simulink model "px4_noGPS1"  (R2022a)
settings: Solver=FixedStepDiscrete  StartTime=0.0  StopTime=inf  FixedStep=0.005  MaxStep=0.000005  RelTol=1e-3  EnableMultiTasking=on
InitFcn:
  | I_x = 0.00478;
  | I_y = 0.00502;
  | I_z = 0.00736;
  | m=1;
  | L=0.11667;
undefined symbols (not defined in the file): alt, cog_rad, dev, DiscIntNeverNeededParam, eph, epv, fix_type, lat, lon, m_to_mm, Main, ms_to_cms, pwm_output0, ref_height, ref_lat, ref_lon, SampleTime, satellites_used, time_utc_usec, vel_d_m_s, vel_e_m_s, vel_m_s, vel_n_m_s, vx, vy, vz, x, y, z
libraries: simulink x26, px4uORBlib x5, px4lib x3, etargetslib x1, sensorgpslib x1, slpidlib x1, sharedtransform x1, px4Sensorslib x1
(part 1 of 3)
settings Model: SimulationMode=external  ExtModeTrigDuration=10  Creator=The MathWorks, Inc.  LastModifiedBy=001
settings SolverCC: AlgebraicLoopSolver=TrustRegion  PositivePriorityOrder=on  AutoInsertRateTranBlk=on
settings DataIOCC: LimitDataPoints=on  MaxDataPoints=10000
settings OptimizationCC: BlockReduction=off  EnhancedBackFolding=on  PassReuseOutputArgsAs=Individual arguments  MaxStackSize=64  OptimizeBlockOrder=speed  DifferentSizesBufferReuse=on  OptimizationCustomize=off  EfficientTunableParamExpr=on
settings DebuggingCC: MultiTaskDSMMsg=none  ParameterTunabilityLossMsg=error  UnconnectedInputMsg=warning  UnconnectedOutputMsg=warning  UnconnectedLineMsg=warning  SFMachineParentedDataDiag=warning  ArithmeticOperatorsInVariantConditions=warning
settings HardwareCC: ProdBitPerPointer=32  ProdBitPerSizeT=32  ProdBitPerPtrDiffT=32  ProdLargestAtomicInteger=Long  ProdLargestAtomicFloat=Double  ProdWordSize=32  ProdLongLongMode=on  ProdHWDeviceType=ARM Compatible->ARM Cortex
settings SFSimCC: SimTargetLang=C++
settings RTWCC: SystemTargetFile=ert.tlc  HardwareBoard=PX4 Pixhawk 1  TLCOptions="-aInlineSetEventsForThisBaseRateFcn=TLC_FALSE -aSuppressMultiTaskScheduler=TLC_FALSE  -aRateBasedStepFcn=0"  TemplateMakefile=ert_default_tmf  GenerateReport=on  Toolchain=GNU Tools for PX4 Autopilots  IncludeHyperlinkInReport=on  LaunchReport=on  TargetLang=C++  GenerateTraceInfo=on  GenerateTraceReport=on  GenerateTraceReportSl=on  GenerateTraceReportSf=on  GenerateTraceReportEml=on
settings CodeAppCC: ForceParamTrailComments=on  IgnoreCustomStorageClasses=off  OperatorAnnotations=on  SimulinkDataObjDesc=on  SFDataObjDesc=on  InsertBlockDesc=on
settings ERTTargetCC: SupportContinuousTime=on  SupportNonInlinedSFcns=on  SupportVariableSizeSignals=on  ExtMode=on  ExtModeMexArgs='127.0.0.1' 1 17725

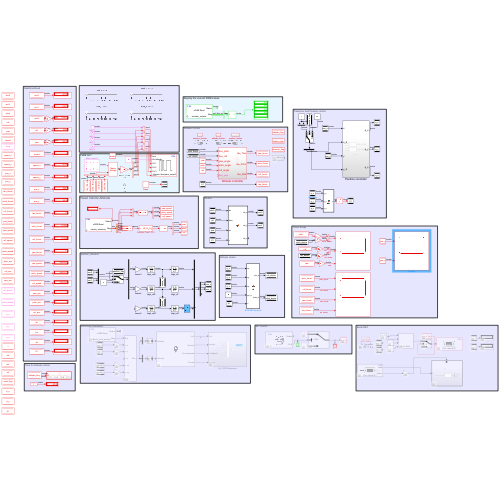
[thumbnail: Simulink's stored preview of the top-level diagram]
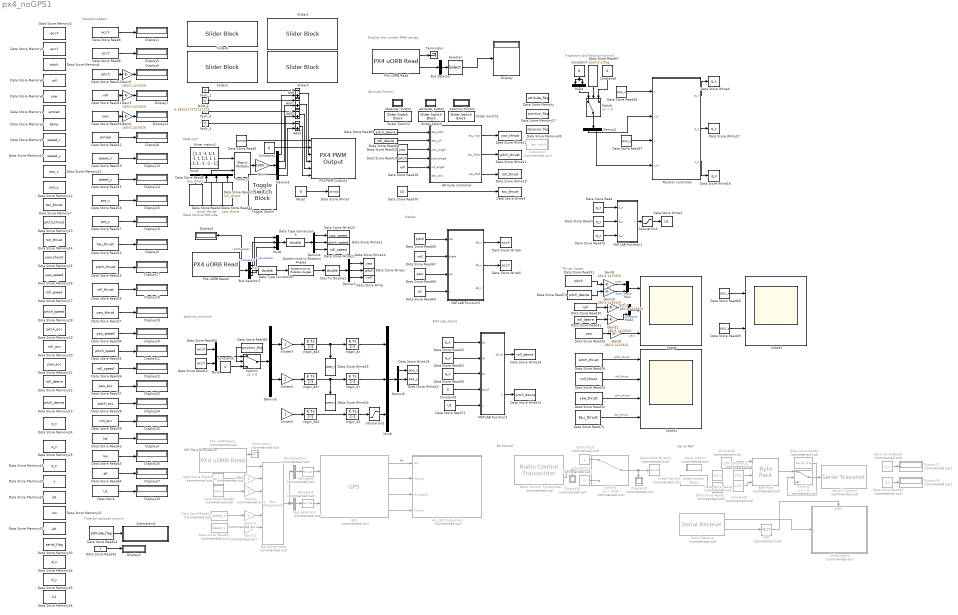
== system px4_noGPS1 ==
  note: Serial R&T
  note: GPS Data Simulation
  note: RC Control
  note: Time for attitude control
  note: position_simulink
  note: Thrust Scope
  note: Attitude Control
  note: DataStoreRead
  note: Display the current PWM values
  note: PWM OUT
  note: Read Vehicle Attitude
  note: Attitude_desire
  note: Trajectory And Position control
  note: GetAcc
  Add{,1..3} (4 alike) : Sum  Inputs=-+  OutDataTypeStr=uint16
  Attitude controller : Subsystem
  Bus Assignment : BusAssignment  Commented=on  AssignedSignals=x,y,z,vx,vy,vz
  Bus Selector : BusSelector  OutputSignals=output  OutputAsBus=on
  Bus Selector1 : BusSelector  Commented=on  OutputSignals=x,y,z  OutputAsBus=on
  Bus Selector2 : BusSelector  OutputSignals=yawspeed,pitchspeed,rollspeed,q
  Bus Selector3 : BusSelector  Commented=on  OutputSignals=vx,vy,vz  OutputAsBus=on
  Byte Pack : etargetslib/Byte Pack  Commented=on  datatypes={'uint8' 'uint8' 'double' 'double'}  byteAlign=1
  Cast To Double1 : DataTypeConversion  OutDataTypeStr=double  SaturateOnIntegerOverflow=off  RndMeth=Floor
  Constant10 : Constant  Commented=on  OutDataTypeStr=boolean
  Constant11 : Constant  Commented=on  Value=0  OutDataTypeStr=boolean
  Constant12 : Constant  Commented=on  Value=10.2  OutDataTypeStr=double
  Constant2 : Constant  Value=0  OutDataTypeStr=boolean
  Constant4 : Constant  Commented=on  Value=10.1  OutDataTypeStr=double
  Constant{5..8} (4 alike) : Constant  Value=0
  Constant9 : Constant  Commented=on  Value=170  OutDataTypeStr=uint8
  "Data Store " : DataStoreRead  DataStoreName=U1  IndexOptions=Index vector (dialog)  Indices=1  OutputSizes=1
  Data Store Memory : DataStoreMemory  DataStoreName=attitude_flag  ReadBeforeWriteMsg=warning  WriteAfterWriteMsg=warning  WriteAfterReadMsg=warning  ShowAdditionalParam=off  OutDataTypeStr=boolean
  Data Store Memory1 : DataStoreMemory  DataStoreName=armed  ReadBeforeWriteMsg=warning  WriteAfterWriteMsg=warning  WriteAfterReadMsg=warning  ShowAdditionalParam=off  OutDataTypeStr=boolean
  Data Store Memory10 : DataStoreMemory  DataStoreName=speed_y  ReadBeforeWriteMsg=warning  WriteAfterWriteMsg=warning  WriteAfterReadMsg=warning  ShowAdditionalParam=off  OutDataTypeStr=double
  Data Store Memory11 : DataStoreMemory  DataStoreName=pos_x  ReadBeforeWriteMsg=warning  WriteAfterWriteMsg=warning  WriteAfterReadMsg=warning  ShowAdditionalParam=off  OutDataTypeStr=double
  Data Store Memory12 : DataStoreMemory  DataStoreName=pos_y  ReadBeforeWriteMsg=warning  WriteAfterWriteMsg=warning  WriteAfterReadMsg=warning  ShowAdditionalParam=off  OutDataTypeStr=double
  Data Store Memory13 : DataStoreMemory  DataStoreName=pitch_thrust  ReadBeforeWriteMsg=warning  WriteAfterWriteMsg=warning  WriteAfterReadMsg=warning  ShowAdditionalParam=off  OutDataTypeStr=double
  Data Store Memory14 : DataStoreMemory  DataStoreName=roll_thrust  ReadBeforeWriteMsg=warning  WriteAfterWriteMsg=warning  WriteAfterReadMsg=warning  ShowAdditionalParam=off  OutDataTypeStr=double
  Data Store Memory15 : DataStoreMemory  DataStoreName=yaw_thrust  ReadBeforeWriteMsg=warning  WriteAfterWriteMsg=warning  WriteAfterReadMsg=warning  ShowAdditionalParam=off  OutDataTypeStr=double
  Data Store Memory16 : DataStoreMemory  DataStoreName=yaw_speed  ReadBeforeWriteMsg=warning  WriteAfterWriteMsg=warning  WriteAfterReadMsg=warning  ShowAdditionalParam=off  OutDataTypeStr=double
  Data Store Memory17 : DataStoreMemory  DataStoreName=roll_speed  ReadBeforeWriteMsg=warning  WriteAfterWriteMsg=warning  WriteAfterReadMsg=warning  ShowAdditionalParam=off  OutDataTypeStr=double
  Data Store Memory18 : DataStoreMemory  DataStoreName=pitch_speed  ReadBeforeWriteMsg=warning  WriteAfterWriteMsg=warning  WriteAfterReadMsg=warning  ShowAdditionalParam=off  OutDataTypeStr=double
  Data Store Memory19 : DataStoreMemory  DataStoreName=pitch_acc  ReadBeforeWriteMsg=warning  WriteAfterWriteMsg=warning  WriteAfterReadMsg=warning  ShowAdditionalParam=off  OutDataTypeStr=double
  Data Store Memory2 : DataStoreMemory  DataStoreName=accX  ReadBeforeWriteMsg=warning  WriteAfterWriteMsg=warning  WriteAfterReadMsg=warning  ShowAdditionalParam=off  OutDataTypeStr=double
  Data Store Memory20 : DataStoreMemory  DataStoreName=roll_acc  ReadBeforeWriteMsg=warning  WriteAfterWriteMsg=warning  WriteAfterReadMsg=warning  ShowAdditionalParam=off  OutDataTypeStr=double
  Data Store Memory21 : DataStoreMemory  DataStoreName=yaw_acc  ReadBeforeWriteMsg=warning  WriteAfterWriteMsg=warning  WriteAfterReadMsg=warning  ShowAdditionalParam=off  OutDataTypeStr=double
  Data Store Memory22 : DataStoreMemory  DataStoreName=roll_desire  ReadBeforeWriteMsg=warning  WriteAfterWriteMsg=warning  WriteAfterReadMsg=warning  ShowAdditionalParam=off  OutDataTypeStr=double
  Data Store Memory23 : DataStoreMemory  DataStoreName=pitch_desire  ReadBeforeWriteMsg=warning  WriteAfterWriteMsg=warning  WriteAfterReadMsg=warning  ShowAdditionalParam=off  OutDataTypeStr=double
  Data Store Memory24 : DataStoreMemory  DataStoreName=q_x  ReadBeforeWriteMsg=warning  WriteAfterWriteMsg=warning  WriteAfterReadMsg=warning  ShowAdditionalParam=off  OutDataTypeStr=double
  Data Store Memory25 : DataStoreMemory  DataStoreName=q_y  ReadBeforeWriteMsg=warning  WriteAfterWriteMsg=warning  WriteAfterReadMsg=warning  ShowAdditionalParam=off  OutDataTypeStr=double
  Data Store Memory26 : DataStoreMemory  DataStoreName=q_z  ReadBeforeWriteMsg=warning  WriteAfterWriteMsg=warning  WriteAfterReadMsg=warning  ShowAdditionalParam=off  OutDataTypeStr=double
  Data Store Memory27 : DataStoreMemory  DataStoreName=position_flag  ReadBeforeWriteMsg=warning  WriteAfterWriteMsg=warning  WriteAfterReadMsg=warning  ShowAdditionalParam=off  OutDataTypeStr=boolean
  Data Store Memory28 : DataStoreMemory  DataStoreName=lat  ReadBeforeWriteMsg=warning  WriteAfterWriteMsg=warning  WriteAfterReadMsg=warning  ShowAdditionalParam=off
  Data Store Memory29 : DataStoreMemory  DataStoreName=t  ReadBeforeWriteMsg=warning  WriteAfterWriteMsg=warning  WriteAfterReadMsg=warning  ShowAdditionalParam=off
  Data Store Memory3 : DataStoreMemory  DataStoreName=accY  ReadBeforeWriteMsg=warning  WriteAfterWriteMsg=warning  WriteAfterReadMsg=warning  ShowAdditionalParam=off  OutDataTypeStr=double
  Data Store Memory30 : DataStoreMemory  DataStoreName=observer_flag  ReadBeforeWriteMsg=warning  WriteAfterWriteMsg=warning  WriteAfterReadMsg=warning  ShowAdditionalParam=off  OutDataTypeStr=boolean
  Data Store Memory31 : DataStoreMemory  DataStoreName=lon  ReadBeforeWriteMsg=warning  WriteAfterWriteMsg=warning  WriteAfterReadMsg=warning  ShowAdditionalParam=off
  Data Store Memory32 : DataStoreMemory  DataStoreName=alt  ReadBeforeWriteMsg=warning  WriteAfterWriteMsg=warning  WriteAfterReadMsg=warning  ShowAdditionalParam=off
  Data Store Memory33 : DataStoreMemory  DataStoreName=serial_flag  ReadBeforeWriteMsg=warning  WriteAfterWriteMsg=warning  WriteAfterReadMsg=warning  ShowAdditionalParam=off
  Data Store Memory34 : DataStoreMemory  DataStoreName=d_x  ReadBeforeWriteMsg=warning  WriteAfterWriteMsg=warning  WriteAfterReadMsg=warning  ShowAdditionalParam=off
  Data Store Memory35 : DataStoreMemory  DataStoreName=d_y  ReadBeforeWriteMsg=warning  WriteAfterWriteMsg=warning  WriteAfterReadMsg=warning  ShowAdditionalParam=off
  Data Store Memory36 : DataStoreMemory  DataStoreName=U1  ReadBeforeWriteMsg=warning  WriteAfterWriteMsg=warning  WriteAfterReadMsg=warning  ShowAdditionalParam=off
  Data Store Memory4 : DataStoreMemory  DataStoreName=pitch  ReadBeforeWriteMsg=warning  WriteAfterWriteMsg=warning  WriteAfterReadMsg=warning  ShowAdditionalParam=off  OutDataTypeStr=double
  Data Store Memory5 : DataStoreMemory  DataStoreName=temp  ReadBeforeWriteMsg=warning  WriteAfterWriteMsg=warning  WriteAfterReadMsg=warning  ShowAdditionalParam=off  OutDataTypeStr=double  Dimensions=5
  Data Store Memory6 : DataStoreMemory  DataStoreName=roll  ReadBeforeWriteMsg=warning  WriteAfterWriteMsg=warning  WriteAfterReadMsg=warning  ShowAdditionalParam=off  OutDataTypeStr=double
  Data Store Memory7 : DataStoreMemory  DataStoreName=tau_thrust  ReadBeforeWriteMsg=warning  WriteAfterWriteMsg=warning  WriteAfterReadMsg=warning  ShowAdditionalParam=off  OutDataTypeStr=double
  Data Store Memory8 : DataStoreMemory  DataStoreName=yaw  ReadBeforeWriteMsg=warning  WriteAfterWriteMsg=warning  WriteAfterReadMsg=warning  ShowAdditionalParam=off  OutDataTypeStr=double
  Data Store Memory9 : DataStoreMemory  DataStoreName=speed_x  ReadBeforeWriteMsg=warning  WriteAfterWriteMsg=warning  WriteAfterReadMsg=warning  ShowAdditionalParam=off  OutDataTypeStr=double
  Data Store Read : DataStoreRead  DataStoreName=q_x  IndexOptions=Index vector (dialog)  Indices=1  OutputSizes=1
  Data Store Read1 : DataStoreRead  Commented=on  DataStoreName=pos_x  IndexOptions=Index vector (dialog)  Indices=1  OutputSizes=1
  Data Store Read{10,14,31,58} (4 alike) : DataStoreRead  DataStoreName=pitch  IndexOptions=Index vector (dialog)  Indices=1  OutputSizes=1
  Data Store Read{11,18,30,67} (4 alike) : DataStoreRead  DataStoreName=roll  IndexOptions=Index vector (dialog)  Indices=1  OutputSizes=1
  Data Store Read12 : DataStoreRead  DataStoreName=armed  IndexOptions=Index vector (dialog)  Indices=1  OutputSizes=1
  Data Store Read13 : DataStoreRead  DataStoreName=tau_thrust  IndexOptions=Index vector (dialog)  Indices=1  OutputSizes=1
  Data Store Read15 : DataStoreRead  DataStoreName=speed_y  IndexOptions=Index vector (dialog)  Indices=1  OutputSizes=1
  Data Store Read16 : DataStoreRead  DataStoreName=pos_x  IndexOptions=Index vector (dialog)  Indices=1  OutputSizes=1
  Data Store Read17 : DataStoreRead  DataStoreName=pos_y  IndexOptions=Index vector (dialog)  Indices=1  OutputSizes=1
  Data Store Read19 : DataStoreRead  DataStoreName=speed_x  IndexOptions=Index vector (dialog)  Indices=1  OutputSizes=1
  Data Store Read2 : DataStoreRead  Commented=on  DataStoreName=pos_y  IndexOptions=Index vector (dialog)  Indices=1  OutputSizes=1
  Data Store Read{20,24,33,66} (4 alike) : DataStoreRead  DataStoreName=yaw  IndexOptions=Index vector (dialog)  Indices=1  OutputSizes=1
  Data Store Read21 : DataStoreRead  DataStoreName=roll_thrust  IndexOptions=Index vector (dialog)  Indices=1  OutputSizes=1
  Data Store Read22 : DataStoreRead  DataStoreName=yaw_thrust  IndexOptions=Index vector (dialog)  Indices=1  OutputSizes=1
  Data Store Read23 : DataStoreRead  DataStoreName=pitch_thrust  IndexOptions=Index vector (dialog)  Indices=1  OutputSizes=1
  Data Store Read25 : DataStoreRead  DataStoreName=pitch_thrust  IndexOptions=Index vector (dialog)  Indices=1  OutputSizes=1
  Data Store Read26 : DataStoreRead  DataStoreName=roll_thrust  IndexOptions=Index vector (dialog)  Indices=1  OutputSizes=1
  Data Store Read27 : DataStoreRead  DataStoreName=yaw_thrust  IndexOptions=Index vector (dialog)  Indices=1  OutputSizes=1
  Data Store Read28 : DataStoreRead  DataStoreName=pitch_thrust  IndexOptions=Index vector (dialog)  Indices=1  OutputSizes=1
  Data Store Read29 : DataStoreRead  DataStoreName=roll_thrust  IndexOptions=Index vector (dialog)  Indices=1  OutputSizes=1
  Data Store Read3 : DataStoreRead  DataStoreName=tau_thrust  IndexOptions=Index vector (dialog)  Indices=1  OutputSizes=1
  Data Store Read32 : DataStoreRead  DataStoreName=yaw_thrust  IndexOptions=Index vector (dialog)  Indices=1  OutputSizes=1
  Data Store Read34 : DataStoreRead  DataStoreName=yaw_speed  IndexOptions=Index vector (dialog)  Indices=1  OutputSizes=1
  Data Store Read35 : DataStoreRead  DataStoreName=pitch_speed  IndexOptions=Index vector (dialog)  Indices=1  OutputSizes=1
  Data Store Read36 : DataStoreRead  DataStoreName=roll_speed  IndexOptions=Index vector (dialog)  Indices=1  OutputSizes=1
  Data Store Read37 : DataStoreRead  DataStoreName=yaw_acc  IndexOptions=Index vector (dialog)  Indices=1  OutputSizes=1
  Data Store Read38 : DataStoreRead  DataStoreName=pitch_acc  IndexOptions=Index vector (dialog)  Indices=1  OutputSizes=1
  Data Store Read39 : DataStoreRead  DataStoreName=roll_acc  IndexOptions=Index vector (dialog)  Indices=1  OutputSizes=1
  Data Store Read4 : DataStoreRead  Commented=on  DataStoreName=serial_flag  IndexOptions=Index vector (dialog)  Indices=1  OutputSizes=1
  Data Store Read40 : DataStoreRead  Commented=on  DataStoreName=d_y  IndexOptions=Index vector (dialog)  Indices=1  OutputSizes=1
  Data Store Read41 : DataStoreRead  DataStoreName=roll_desire  IndexOptions=Index vector (dialog)  Indices=1  OutputSizes=1
  Data Store Read42 : DataStoreRead  DataStoreName=lat  IndexOptions=Index vector (dialog)  Indices=1  OutputSizes=1
  Data Store Read43 : DataStoreRead  DataStoreName=lon  IndexOptions=Index vector (dialog)  Indices=1  OutputSizes=1
  Data Store Read44 : DataStoreRead  DataStoreName=alt  IndexOptions=Index vector (dialog)  Indices=1  OutputSizes=1
  Data Store Read45 : DataStoreRead  DataStoreName=q_x  IndexOptions=Index vector (dialog)  Indices=1  OutputSizes=1
  Data Store Read46 : DataStoreRead  DataStoreName=pos_x  IndexOptions=Index vector (dialog)  Indices=1  OutputSizes=1
  Data Store Read47 : DataStoreRead  DataStoreName=pos_y  IndexOptions=Index vector (dialog)  Indices=1  OutputSizes=1
  Data Store Read48 : DataStoreRead  DataStoreName=pos_x  IndexOptions=Index vector (dialog)  Indices=1  OutputSizes=1
  Data Store Read49 : DataStoreRead  DataStoreName=pos_y  IndexOptions=Index vector (dialog)  Indices=1  OutputSizes=1
  Data Store Read5 : DataStoreRead  Commented=on  DataStoreName=d_x  IndexOptions=Index vector (dialog)  Indices=1  OutputSizes=1
  Data Store Read50 : DataStoreRead  DataStoreName=accX  IndexOptions=Index vector (dialog)  Indices=1  OutputSizes=1
  Data Store Read51 : DataStoreRead  DataStoreName=accY  IndexOptions=Index vector (dialog)  Indices=1  OutputSizes=1
  Data Store Read52 : DataStoreRead  DataStoreName=q_y  IndexOptions=Index vector (dialog)  Indices=1  OutputSizes=1
  Data Store Read53 : DataStoreRead  DataStoreName=position_flag  IndexOptions=Index vector (dialog)  Indices=1  OutputSizes=1
  Data Store Read54 : DataStoreRead  DataStoreName=attitude_flag  IndexOptions=Index vector (dialog)  Indices=1  OutputSizes=1
  Data Store Read55 : DataStoreRead  DataStoreName=t  IndexOptions=Index vector (dialog)  Indices=1  OutputSizes=1
  Data Store Read56 : DataStoreRead  DataStoreName=q_z  IndexOptions=Index vector (dialog)  Indices=1  OutputSizes=1
  Data Store Read57 : DataStoreRead  DataStoreName=position_flag  IndexOptions=Index vector (dialog)  Indices=1  OutputSizes=1
  Data Store Read59 : DataStoreRead  Commented=on  DataStoreName=pos_x  IndexOptions=Index vector (dialog)  Indices=1  OutputSizes=1
  Data Store Read6 : DataStoreRead  DataStoreName=armed  IndexOptions=Index vector (dialog)  Indices=1  OutputSizes=1
  Data Store Read60 : DataStoreRead  Commented=on  DataStoreName=pos_y  IndexOptions=Index vector (dialog)  Indices=1  OutputSizes=1
  Data Store Read61 : DataStoreRead  Commented=on  DataStoreName=speed_x  IndexOptions=Index vector (dialog)  Indices=1  OutputSizes=1
  Data Store Read62 : DataStoreRead  Commented=on  DataStoreName=speed_y  IndexOptions=Index vector (dialog)  Indices=1  OutputSizes=1
  Data Store Read63 : DataStoreRead  DataStoreName=U1  IndexOptions=Index vector (dialog)  Indices=1  OutputSizes=1
  Data Store Read68 : DataStoreRead  DataStoreName=roll_desire  IndexOptions=Index vector (dialog)  Indices=1  OutputSizes=1
  Data Store Read69 : DataStoreRead  DataStoreName=pitch_desire  IndexOptions=Index vector (dialog)  Indices=1  OutputSizes=1
  Data Store Read7 : DataStoreRead  DataStoreName=q_y  IndexOptions=Index vector (dialog)  Indices=1  OutputSizes=1
  Data Store Read70 : DataStoreRead  DataStoreName=U1  IndexOptions=Index vector (dialog)  Indices=1  OutputSizes=1
  Data Store Read71 : DataStoreRead  DataStoreName=U1  IndexOptions=Index vector (dialog)  Indices=1  OutputSizes=1
  Data Store Read73 : DataStoreRead  DataStoreName=tau_thrust  IndexOptions=Index vector (dialog)  Indices=1  OutputSizes=1
  Data Store Read74 : DataStoreRead  DataStoreName=pitch_desire  IndexOptions=Index vector (dialog)  Indices=1  OutputSizes=1
  Data Store Read75 : DataStoreRead  DataStoreName=q_z  IndexOptions=Index vector (dialog)  Indices=1  OutputSizes=1
  Data Store Read8 : DataStoreRead  DataStoreName=accX  IndexOptions=Index vector (dialog)  Indices=1  OutputSizes=1
  Data Store Read9 : DataStoreRead  DataStoreName=accY  IndexOptions=Index vector (dialog)  Indices=1  OutputSizes=1
  Data Store Write : DataStoreWrite  DataStoreName=roll  IndexOptions=Index vector (dialog)  Indices=1  OutputSizes=1
  Data Store Write1 : DataStoreWrite  DataStoreName=pitch  IndexOptions=Index vector (dialog)  Indices=1  OutputSizes=1
  Data Store Write10 : DataStoreWrite  DataStoreName=yaw  IndexOptions=Index vector (dialog)  Indices=1  OutputSizes=1
  Data Store Write11 : DataStoreWrite  DataStoreName=yaw_thrust  IndexOptions=Index vector (dialog)  Indices=1  OutputSizes=1
  Data Store Write12 : DataStoreWrite  DataStoreName=pitch_thrust  IndexOptions=Index vector (dialog)  Indices=1  OutputSizes=1
  Data Store Write13 : DataStoreWrite  DataStoreName=roll_thrust  IndexOptions=Index vector (dialog)  Indices=1  OutputSizes=1
  Data Store Write14 : DataStoreWrite  DataStoreName=roll_desire  IndexOptions=Index vector (dialog)  Indices=1  OutputSizes=1
  Data Store Write15 : DataStoreWrite  DataStoreName=pitch_desire  IndexOptions=Index vector (dialog)  Indices=1  OutputSizes=1
  Data Store Write16 : DataStoreWrite  Commented=on  DataStoreName=armed  IndexOptions=Index vector (dialog)  Indices=1  OutputSizes=1
  Data Store Write17 : DataStoreWrite  DataStoreName=q_y  IndexOptions=Index vector (dialog)  Indices=1  OutputSizes=1
  Data Store Write18 : DataStoreWrite  DataStoreName=q_z  IndexOptions=Index vector (dialog)  Indices=1  OutputSizes=1
  Data Store Write19 : DataStoreWrite  DataStoreName=pos_x  IndexOptions=Index vector (dialog)  Indices=1  OutputSizes=1
  Data Store Write2 : DataStoreWrite  DataStoreName=U1  IndexOptions=Index vector (dialog)  Indices=1  OutputSizes=1
  Data Store Write20 : DataStoreWrite  DataStoreName=yaw_speed  IndexOptions=Index vector (dialog)  Indices=1  OutputSizes=1
  Data Store Write21 : DataStoreWrite  DataStoreName=pitch_speed  IndexOptions=Index vector (dialog)  Indices=1  OutputSizes=1
  Data Store Write22 : DataStoreWrite  DataStoreName=roll_speed  IndexOptions=Index vector (dialog)  Indices=1  OutputSizes=1
  Data Store Write23 : DataStoreWrite  DataStoreName=pos_y  IndexOptions=Index vector (dialog)  Indices=1  OutputSizes=1
  Data Store Write24 : DataStoreWrite  DataStoreName=speed_y  IndexOptions=Index vector (dialog)  Indices=1  OutputSizes=1
  Data Store Write25 : DataStoreWrite  DataStoreName=speed_x  IndexOptions=Index vector (dialog)  Indices=1  OutputSizes=1
  Data Store Write4 : DataStoreWrite  DataStoreName=q_x  IndexOptions=Index vector (dialog)  Indices=1  OutputSizes=1
  Data Store Write5 : DataStoreWrite  DataStoreName=accY  IndexOptions=Index vector (dialog)  Indices=1  OutputSizes=1
  Data Store Write6 : DataStoreWrite  DataStoreName=accX  IndexOptions=Index vector (dialog)  Indices=1  OutputSizes=1
  Data Store Write7 : DataStoreWrite  DataStoreName=armed  IndexOptions=Index vector (dialog)  Indices=1  OutputSizes=1
  Data Store Write9 : DataStoreWrite  DataStoreName=tau_thrust  IndexOptions=Index vector (dialog)  Indices=1  OutputSizes=1
  Data Type Conversion1 : DataTypeConversion  OutDataTypeStr=double  SaturateOnIntegerOverflow=off  RndMeth=Floor
  Data Type Conversion3 : DataTypeConversion  OutDataTypeStr=double  SaturateOnIntegerOverflow=off  RndMeth=Floor
  Demux1 : Demux  Outputs=3
  Demux2 : Demux  Outputs=2
  Demux3 : Demux
  Demux4 : Demux  Outputs=3
  Demux5 : Demux  Outputs=2
  Demux6 : Demux  Outputs=3
  Display{,1..9,12..27,30} (27 alike) : Display
  Display{10..11,28..29} (4 alike) : Display  Commented=on
  GPS : sensorgpslib/GPS  Commented=on  DispRefFrame=NED  PositionInputFormat=Local  ReferenceLocation=[ref_lat ref_lon ref_height]  HorizontalPositionAccuracy=0.01  VerticalPositionAccuracy=0.01  VelocityAccuracy=0.01  DecayFactor=0.999  SeedDouble=67  SimulateUsing=Interpreted execution
      settings: SourceProductBaseCode=TF,NV,UV
  Gain{,12..14} (4 alike) : Gain  Commented=on  OutDataTypeStr=single
  Gain{3,5..11} (8 alike) : Gain  Gain=180/3.1415926
  Gain4 : Gain  Gain=1000  OutDataTypeStr=uint16
  HIL_GPS Subsystem : Subsystem  Commented=on
  Intgrt_dX : DiscreteIntegrator  gainval=1  SampleTime=-1  ICPrevOutput=DiscIntNeverNeededParam  ICPrevScaledInput=DiscIntNeverNeededParam
  Intgrt_dY : DiscreteIntegrator  gainval=1  SampleTime=-1  ICPrevOutput=DiscIntNeverNeededParam  ICPrevScaledInput=DiscIntNeverNeededParam
  Intgrt_dZ : DiscreteIntegrator  gainval=1  SampleTime=-1  LowerSaturationLimit=0  ICPrevOutput=DiscIntNeverNeededParam  ICPrevScaledInput=DiscIntNeverNeededParam
  Intgrt_ddX : DiscreteIntegrator  gainval=1  SampleTime=-1  ICPrevOutput=DiscIntNeverNeededParam  ICPrevScaledInput=DiscIntNeverNeededParam
  Intgrt_ddY : DiscreteIntegrator  gainval=1  SampleTime=-1  ICPrevOutput=DiscIntNeverNeededParam  ICPrevScaledInput=DiscIntNeverNeededParam
  Intgrt_ddZ : DiscreteIntegrator  gainval=1  SampleTime=-1  ICPrevOutput=DiscIntNeverNeededParam  ICPrevScaledInput=DiscIntNeverNeededParam
  MATLAB Function1 : MATLAB Function  TreatAsAtomicUnit=on
  MATLAB Function3 : MATLAB Function  TreatAsAtomicUnit=on
  MATLAB Function5 : MATLAB Function  TreatAsAtomicUnit=on
  Mixer matrix1 : Constant  Value=[1 1 -1 1;1 -1 1 1;1 1 1 -1;1 -1 -1 -1]  OutDataTypeStr=Inherit: Inherit via back propagation
  Mux{,2,4..5} (4 alike) : Mux  Inputs=2
  Mux3 : Mux
  Mux6 : Mux  Inputs=3
  Mux8 : Mux  Inputs=3
  NOT : Logic  Commented=on  Operator=NOT  IconShape=distinctive  AllPortsSameDT=off  OutDataTypeStr=boolean
  PX4 PWM Output1 : px4lib/PX4 PWM Output  pwmDevice=Main (/dev/pwm_output0)  pwmChannel1_=on  pwmChannel2_=on  pwmChannel3_=on  pwmChannel4_=on  pwmChannel5_=off  pwmChannel6_=off  pwmChannel7_=off  pwmChannel8_=off  forceTerminateFailsafe=off  outputErrorStatus=off
      settings: SourceProductBaseCode=PX4AUTOPILOTS
  PX4 uORB Read : px4uORBlib/PX4 uORB Read  uORBTopic=actuator_outputs  selectInstance=actuator_outputs  SampleTime=0.01  BlockingMode=off  BlockTimeout=1e-3
      settings: SourceProductBaseCode=PX4AUTOPILOTS
  PX4 uORB Read1 : px4uORBlib/PX4 uORB Read  Commented=on  uORBTopic=vehicle_local_position  selectInstance=vehicle_local_position  SampleTime=-1  BlockingMode=off  BlockTimeout=1e-3
      settings: SourceProductBaseCode=PX4AUTOPILOTS
  PX4 uORB Read2 : px4uORBlib/PX4 uORB Read  uORBTopic=vehicle_odometry  selectInstance=vehicle_odometry  SampleTime=0.005  BlockingMode=off  BlockTimeout=1e-3
      settings: SourceProductBaseCode=PX4AUTOPILOTS
  Position controller : Subsystem
  Product2 : Product  Multiplication=Matrix(*)  RndMeth=Zero
  Quaternions to Rotation Angles : sharedtransform/Quaternions to Rotation Angles  rotationOrder=ZYX  aMode=aMode
      settings: SourceProductBaseCode=AE,PW,DR,MT,VE
  Radio Control Transmitter : px4Sensorslib/Radio Control Transmitter  Commented=on  channel1=off  channel2=off  channel3=off  channel4=off  channel5=off  channel6=off  channel7=off  channel8=on  channel_count=off  rssi=off  rc_input_source=off  timestamp_last_signal=off  time_stamp=off  sampleTime=0.005  BlockingMode=off  BlockTimeout=5
      settings: SourceProductBaseCode=PX4AUTOPILOTS
  Reset : Constant  Value=0  OutDataTypeStr=boolean  SampleTime=-1
      settings: OpenFcn=|
      | if strcmp('0',get_param(gcb, 'Value'))                        set_param(gcb, 'Value', '1');
      | else
      |             set_param(gcb, 'Value', '0');
      | end
  Reshape1 : Reshape  Commented=on  OutputDimensionality=Row vector (2-D)
  Reshape3 : Reshape  Commented=on  OutputDimensionality=Row vector (2-D)
  Saturation1 : Saturate  UpperLimit=inf  LowerLimit=0
  Saturation2 : Saturate  UpperLimit=1.5  LowerLimit=1
  Scope : Scope  NumInputPorts=3
  Scope1 : Scope  NumInputPorts=4
  Scope2 : Scope  NumInputPorts=2
  Selector : Selector  InputPortWidth=16  IndexOptions=Select all  Indices=[1 4]  OutputSizes=1
  Serial Receive : px4lib/Serial Receive  Commented=on  SCIModule=/dev/ttyS1  DataType=uint8  DataLength=36  OutputStatus=on  SampleTime=-1  BlockingMode=off  PartialData=off  Timeout=5
      settings: SourceProductBaseCode=PX4AUTOPILOTS
  Serial Transmit : px4lib/Serial Transmit  Commented=on  SCIModule=/dev/ttyS1
      settings: SourceProductBaseCode=PX4AUTOPILOTS
  Slider Switch : SliderSwitchBlock
      settings: Values={{'Off', 'On'}, [0 1]}
  Slider Switch1 : SliderSwitchBlock
      settings: Values={{'Off', 'On'}, [0 1]}
  Slider Switch2 : SliderSwitchBlock
      settings: Values={{'Off', 'On'}, [0 1]}
  Slider Switch3 : SliderSwitchBlock  Commented=on
      settings: Values={{'Off', 'On'}, [0 1]}
  Slider{1..3,6} (4 alike) : SliderBlock  ScaleMax=200
  Subsystem : Subsystem  Commented=on
  Subsystem1 : Subsystem
  Subsystem2 : Subsystem  Commented=on
  Switch : Switch  Criteria=u2 > Threshold  SaturateOnIntegerOverflow=off  InputSameDT=off
  Switch1 : Switch  Criteria=u2 > Threshold  SaturateOnIntegerOverflow=off  InputSameDT=off
  Switch2 : Switch  Commented=on  Criteria=u2 > Threshold  SaturateOnIntegerOverflow=off  InputSameDT=off
  Switch3 : Switch  Commented=on  Criteria=u2 > Threshold  Threshold=1500  SaturateOnIntegerOverflow=off  InputSameDT=off
  Terminator : Terminator
  Terminator1 : Terminator  Commented=on
  Toggle Switch : ToggleSwitchBlock
      settings: Values={{'Off', 'On'}, [0 1]}
  attitude_button : Subsystem
  fault_1 : Constant  Value=0
  fault_2 : Constant  Value=0.3835227272727273
  fault_3 : Constant  Value=0
  fault_4 : Constant  Value=0
  observer_button : Subsystem
  position_button : Subsystem
  serial_button : Subsystem  Commented=on
  slower3 : Gain
  slower4 : Gain
  slower5 : Gain
  wires:
  PX4 uORB Read/1 -> Terminator/1
  PX4 uORB Read/2 -> Bus Selector/1
  Bus Selector/1 -> Selector/1
  Selector/1 -> Display/1
  PX4 uORB Read2/1 -> Display2/1
  Quaternions to Rotation Angles/1 -> Cast To Double1/1
  Data Type Conversion1/1 -> Quaternions to Rotation Angles/1
  Bus Selector2/4 -> Data Type Conversion1/1  "<q>"
  PX4 uORB Read2/2 -> Bus Selector2/1
  Demux1/3 -> Data Store Write/1
  Demux1/2 -> Data Store Write1/1
  Cast To Double1/1 -> Demux1/1
  Data Store Read8/1 -> Display1/1
  Data Store Read9/1 -> Display5/1
  Data Store Read12/1 -> Display8/1
  Data Store Read19/1 -> Display13/1
  Data Store Read16/1 -> Display15/1
  Data Store Read17/1 -> Display16/1
  Data Store Read15/1 -> Display14/1
  Data Store Read13/1 -> Display9/1
  Mux3/1 -> Product2/2
  Product2/1 -> Gain4/1
  Gain4/1 -> Demux3/1
  Data Store Read3/1 -> Mux3/1
  Data Store Read6/1 -> PX4 PWM Output1/1
  Data Store Read11/1 -> Gain3/1
  Gain3/1 -> Display7/1
  Data Store Read10/1 -> Gain5/1
  Gain5/1 -> Display6/1
  Data Store Read14/1 -> Attitude controller/4(pitch_angle)
  Data Store Read18/1 -> Attitude controller/5("roll_angle ")
  Demux1/1 -> Data Store Write10/1
  Data Store Read20/1 -> Attitude controller/3(yaw_angle)
  Attitude controller/1(tau_Yaw) -> Data Store Write11/1
  Attitude controller/2(tau_Pitch) -> Data Store Write12/1
  Attitude controller/3(tau_Roll) -> Data Store Write13/1
  Data Store Read22/1 -> Mux3/4
  Data Store Read25/1 -> Display17/1
  Data Store Read26/1 -> Display18/1
  Data Store Read27/1 -> Display19/1
  Data Store Read28/1 -> Scope1/1  "pitch_thrust"
  Data Store Read24/1 -> Gain6/1
  Gain6/1 -> Display12/1
  Gain8/1 -> Mux/1  "pitch"
  Data Store Read31/1 -> Gain8/1
  Data Store Read30/1 -> Gain7/1
  Data Store Read29/1 -> Scope1/2  "roll_thrust"
  Data Store Read33/1 -> Gain9/1
  Gain9/1 -> Scope/3  "yaw"
  Data Store Read32/1 -> Scope1/3  "yaw_thrust"
  Data Store Read34/1 -> Display20/1
  Data Store Read35/1 -> Display21/1
  Data Store Read36/1 -> Display22/1
  Data Store Read38/1 -> Display24/1
  Data Store Read39/1 -> Display25/1
  Data Store Read37/1 -> Display23/1
  Mux6/1 -> Data Type Conversion3/1
  Data Type Conversion3/1 -> Demux4/1
  Demux4/1 -> Data Store Write20/1
  Demux4/2 -> Data Store Write21/1
  Demux4/3 -> Data Store Write22/1
  Constant2/1 -> PX4 PWM Output1/2
  Mixer matrix1/1 -> Product2/1
  Mux/1 -> Scope/1
  Mux2/1 -> Scope/2
  Gain7/1 -> Mux2/1  "roll"
  Data Store Read48/1 -> Scope2/1
  Data Store Read49/1 -> Scope2/2
  Data Store Read54/1 -> Subsystem1/Enable
  Data Store Read55/1 -> Display3/1
  Data Store Read23/1 -> Mux3/2
  Data Store Read21/1 -> Mux3/3
  fault_1/1 -> Add/1
  fault_2/1 -> Add1/1
  fault_3/1 -> Add2/1
  fault_4/1 -> Add3/1
  Demux3/1 -> Add/2
  Demux3/2 -> Add1/2
  Demux3/3 -> Add2/2
  Demux3/4 -> Add3/2
  Add/1 -> PX4 PWM Output1/3
  Add1/1 -> PX4 PWM Output1/4
  Add2/1 -> PX4 PWM Output1/5
  Add3/1 -> PX4 PWM Output1/6
  Gain10/1 -> Mux/2  "pitch_desire"
  Gain11/1 -> Mux2/2  "roll_desire"
  Constant10/1 -> Switch3/1
  Constant11/1 -> Switch3/3
  Switch3/1 -> Data Store Write16/1, Display28/1
  Bus Selector2/1 -> Mux6/1  "<yawspeed>"
  Bus Selector2/2 -> Mux6/2  "<pitchspeed>"
  Bus Selector2/3 -> Mux6/3  "<rollspeed>"
  GPS/4 -> HIL_GPS Subsystem/4(Course)
  GPS/1 -> HIL_GPS Subsystem/1(LLA)  "lla"
  Reshape3/1 -> GPS/1
  GPS/3 -> HIL_GPS Subsystem/3(GndSpeed)
  GPS/2 -> HIL_GPS Subsystem/2(Velocity)
  Bus Selector3/1 -> Reshape1/1
  Bus Selector1/1 -> Reshape3/1
  Reshape1/1 -> GPS/2
  PX4 uORB Read1/2 -> Bus Assignment/1
  Data Store Read59/1 -> Gain/1
  Data Store Read60/1 -> Gain12/1
  Data Store Read61/1 -> Gain13/1
  Data Store Read62/1 -> Gain14/1
  Bus Assignment/1 -> Bus Selector3/1, Bus Selector1/1
  PX4 uORB Read1/1 -> Terminator1/1
  Gain/1 -> Bus Assignment/2
  Gain12/1 -> Bus Assignment/3
  Gain13/1 -> Bus Assignment/5
  Gain14/1 -> Bus Assignment/6
  Demux5/2 -> slower4/1
  Data Store Read50/1 -> Mux5/1
  Data Store Read53/1 -> Switch1/2
  Mux5/1 -> Switch1/1
  Data Store Read51/1 -> Mux5/2
  Demux5/1 -> slower3/1
  Switch1/1 -> Demux5/1
  Intgrt_dY/1 -> Mux8/2
  slower4/1 -> Intgrt_ddY/1
  Demux6/1 -> Data Store Write19/1
  Demux6/2 -> Data Store Write23/1
  Intgrt_ddZ/1 -> Intgrt_dZ/1
  slower5/1 -> Intgrt_ddZ/1
  Intgrt_ddX/1 -> Data Store Write25/1, Intgrt_dX/1
  Intgrt_dZ/1 -> Saturation1/1
  Constant5/1 -> Switch1/3
  slower3/1 -> Intgrt_ddX/1
  Mux8/1 -> Demux6/1
  Intgrt_dX/1 -> Mux8/1
  Saturation1/1 -> Mux8/3
  Intgrt_ddY/1 -> Data Store Write24/1, Intgrt_dY/1
  Data Store Read43/1 -> Display26/1
  Data Store Read42/1 -> Display4/1
  Data Store Read44/1 -> Display27/1
  Radio Control Transmitter/2 -> Switch3/2, Display10/1
  Serial Receive/2 -> NOT/1
  Switch2/1 -> Serial Transmit/1
  Constant9/1 -> Byte Pack/2, Byte Pack/1
  Data Store Read4/1 -> Switch2/2
  Constant4/1 -> Byte Pack/4
  Constant12/1 -> Byte Pack/3
  Data Store Read5/1 -> Display11/1
  Data Store Read40/1 -> Display29/1
  Byte Pack/1 -> Switch2/1
  Serial Receive/1 -> Subsystem2/1(u)
  NOT/1 -> Subsystem2/Enable
  Data Store Read52/1 -> MATLAB Function3/2(qy)
  MATLAB Function3/1(phi_d) -> Data Store Write14/1
  MATLAB Function3/2(theta_d) -> Data Store Write15/1
  Data Store Read56/1 -> MATLAB Function3/3(qz)
  Data Store Read71/1 -> MATLAB Function3/5(u)
  Data Store Read45/1 -> MATLAB Function3/1(qx)
  Constant6/1 -> MATLAB Function3/4(psi_d)
  Demux2/2 -> Position controller/4(y_d)
  Switch/1 -> Demux2/1
  Constant8/1 -> Switch/3
  Data Store Read47/1 -> Position controller/3(y)
  Position controller/3(q_z) -> Data Store Write18/1
  Demux2/1 -> Position controller/2(x_d)
  Data Store Read57/1 -> Switch/2
  Constant7/1 -> Mux4/1, Mux4/2
  Mux4/1 -> Switch/1
  Data Store Read46/1 -> Position controller/1(x)
  Position controller/2(q_y) -> Data Store Write17/1
  Position controller/1(q_x) -> Data Store Write4/1
  MATLAB Function5/1(dd_x) -> Data Store Write6/1
  MATLAB Function5/2(dd_y) -> Data Store Write5/1
  Data Store Read58/1 -> MATLAB Function5/1(phi)
  Data Store Read67/1 -> MATLAB Function5/2(theta)
  Data Store Read63/1 -> MATLAB Function5/4(u)
  Data Store Read66/1 -> MATLAB Function5/3(psi)
  Data Store Read73/1 -> Scope1/4  "tau_thrust"
  Data Store Read41/1 -> Gain11/1
  Data Store Read74/1 -> Gain10/1
  Reset/1 -> Data Store Write7/1
  Data Store Read68/1 -> Attitude controller/2(des_roll)
  Data Store Read69/1 -> Attitude controller/1(des_pitch)
  Data Store Read/1 -> MATLAB Function1/1(q_x)
  Data Store Read7/1 -> MATLAB Function1/2(q_y)
  Data Store Read75/1 -> MATLAB Function1/3(q_z)
  MATLAB Function1/1(u) -> Saturation2/1
  Saturation2/1 -> Data Store Write2/1
  "Data Store "/1 -> Display30/1
  Data Store Read70/1 -> Data Store Write9/1

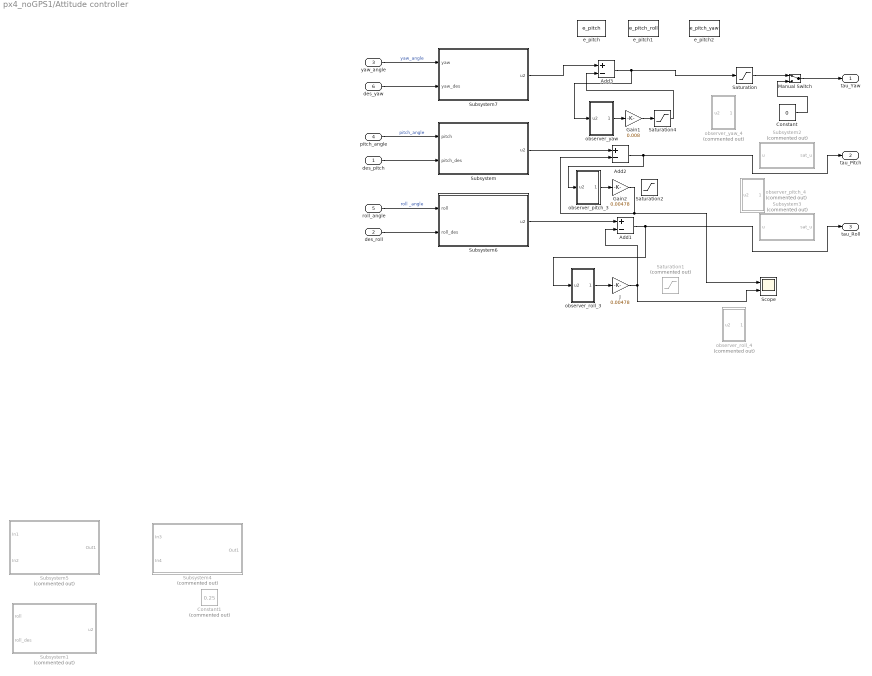
== system px4_noGPS1/Attitude controller ==
  des_pitch : Inport
  des_roll : Inport  Port=2
  yaw_angle : Inport  Port=3
  pitch_angle : Inport  Port=4
  "roll_angle " : Inport  Port=5
  des_yaw : Inport  Port=6
  Add1 : Sum  Inputs=+-
  Add2 : Sum  Inputs=+-
  Add3 : Sum  Inputs=+-
  Constant : Constant  Value=0
  Constant1 : Constant  Commented=on  Value=0.25
  Gain1 : Gain  Gain=0.008
  Gain2 : Gain  Gain=0.00478
  J : Gain  Gain=0.00478
  Manual Switch : ManualSwitch
  Saturation : Saturate  UpperLimit=0.1  LowerLimit=-0.1
  Saturation1 : Saturate  Commented=on  UpperLimit=0.2
  Saturation2 : Saturate  UpperLimit=0.2
  Saturation4 : Saturate  UpperLimit=0.2
  Scope : Scope  NumInputPorts=2
  Subsystem : Subsystem
  Subsystem1 : Subsystem  Commented=on
  Subsystem2 : Subsystem  Commented=on
  Subsystem3 : Subsystem  Commented=on
  Subsystem4 : Subsystem  Commented=on  mask{c=1, g=1}
      mask prompts: c "gain_1"; g "gain_2"
  Subsystem5 : Subsystem  Commented=on  mask{c=1, g=1}
      mask prompts: c "gain_1"; g "gain_2"
  Subsystem6 : Subsystem
  Subsystem7 : Subsystem
  e_pitch : DataStoreMemory  DataStoreName=e_pitch  ReadBeforeWriteMsg=warning  WriteAfterWriteMsg=warning  WriteAfterReadMsg=warning  ShowAdditionalParam=off
  e_pitch1 : DataStoreMemory  DataStoreName=e_pitch_roll  ReadBeforeWriteMsg=warning  WriteAfterWriteMsg=warning  WriteAfterReadMsg=warning  ShowAdditionalParam=off
  e_pitch2 : DataStoreMemory  DataStoreName=e_pitch_yaw  ReadBeforeWriteMsg=warning  WriteAfterWriteMsg=warning  WriteAfterReadMsg=warning  ShowAdditionalParam=off
  observer_pitch_3 : Subsystem
  observer_pitch_4 : Subsystem  Commented=on
  observer_roll_3 : Subsystem
  observer_roll_4 : Subsystem  Commented=on
  observer_yaw : Subsystem
  observer_yaw_4 : Subsystem  Commented=on
  tau_Yaw : Outport
  tau_Pitch : Outport  Port=2
  tau_Roll : Outport  Port=3
  wires:
  Saturation/1 -> Manual Switch/1
  Constant/1 -> Manual Switch/2
  Subsystem/1(u2) -> Add2/1
  Add2/1 -> observer_pitch_3/1(u2), tau_Pitch/1
  des_pitch/1 -> Subsystem/2(pitch_des)
  pitch_angle/1 -> Subsystem/1(pitch)  "pitch_angle"
  Manual Switch/1 -> tau_Yaw/1
  "roll_angle "/1 -> Subsystem6/1(roll)  "roll _angle"
  des_roll/1 -> Subsystem6/2(roll_des)
  yaw_angle/1 -> Subsystem7/1(yaw)  "yaw_angle"
  des_yaw/1 -> Subsystem7/2(yaw_des)
  Add1/1 -> observer_roll_3/1(u2), tau_Roll/1
  Subsystem6/1(u2) -> Add1/1
  Saturation4/1 -> Add3/2
  Gain1/1 -> Saturation4/1
  Add3/1 -> observer_yaw/1(u2), Saturation/1
  Subsystem7/1(u2) -> Add3/1
  observer_yaw/1(Out1) -> Gain1/1
  observer_roll_3/1(Out1) -> J/1
  observer_pitch_3/1(Out1) -> Gain2/1
  J/1 -> Scope/2, Add1/2
  Gain2/1 -> Scope/1, Add2/2

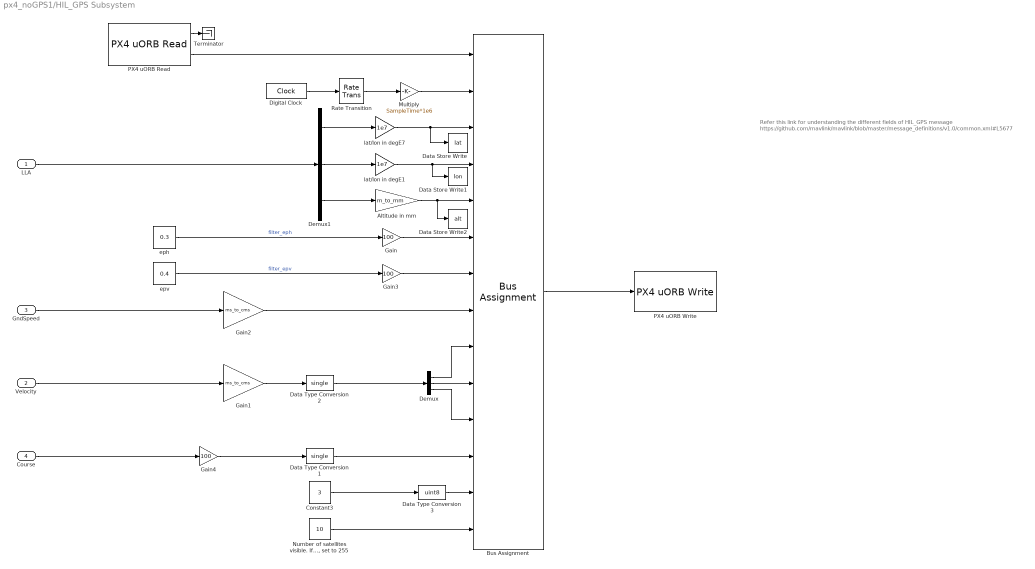
== system px4_noGPS1/HIL_GPS Subsystem ==
  note: Refer this link for understanding the different fields of HIL_GPS message https://github.com/mavlink/mavlink/blob/master/message_definitions/v1.0/common.xml#L5677
  LLA : Inport
  Velocity : Inport  Port=2
  GndSpeed : Inport  Port=3
  Course : Inport  Port=4
  Altitude in mm : Gain  Gain=m_to_mm  OutDataTypeStr=Inherit: Inherit via back propagation
  Bus Assignment : BusAssignment  AssignedSignals=time_utc_usec,lat,lon,alt,eph,epv,vel_m_s,vel_n_m_s,vel_e_m_s,vel_d_m_s,cog_rad,fix_type,satellites_used
  Constant3 : Constant  Value=3  OutDataTypeStr=Inherit: Inherit via back propagation  SampleTime=-1
  Data Store Write : DataStoreWrite  DataStoreName=lat  IndexOptions=Index vector (dialog)  Indices=1  OutputSizes=1
  Data Store Write1 : DataStoreWrite  DataStoreName=lon  IndexOptions=Index vector (dialog)  Indices=1  OutputSizes=1
  Data Store Write2 : DataStoreWrite  DataStoreName=alt  IndexOptions=Index vector (dialog)  Indices=1  OutputSizes=1
  Data Type Conversion1 : DataTypeConversion  OutDataTypeStr=single  SaturateOnIntegerOverflow=off  RndMeth=Floor
  Data Type Conversion2 : DataTypeConversion  OutDataTypeStr=single  SaturateOnIntegerOverflow=off  RndMeth=Floor
  Data Type Conversion3 : DataTypeConversion  OutDataTypeStr=uint8  SaturateOnIntegerOverflow=off  RndMeth=Floor
  Demux : Demux  Outputs=3
  Demux1 : Demux  Outputs=3
  Digital Clock : DigitalClock  SampleTime=-1
  Gain : Gain  Gain=100  OutDataTypeStr=Inherit: Inherit via back propagation
  Gain1 : Gain  Gain=ms_to_cms
  Gain2 : Gain  Gain=ms_to_cms  OutDataTypeStr=single
  Gain3 : Gain  Gain=100  OutDataTypeStr=Inherit: Inherit via back propagation
  Gain4 : Gain  Gain=100
  Multiply : Gain  Gain=SampleTime*1e6  OutDataTypeStr=Inherit: Inherit via back propagation
  "Number of satellites visible. If unknown, set to 255" : Constant  Value=10  OutDataTypeStr=Inherit: Inherit via back propagation  SampleTime=-1
  PX4 uORB Read : px4uORBlib/PX4 uORB Read  uORBTopic=vehicle_gps_position  selectInstance=vehicle_gps_position  SampleTime=-1  BlockingMode=off  BlockTimeout=1e-3
      settings: SourceProductBaseCode=PX4AUTOPILOTS
  PX4 uORB Write : px4uORBlib/PX4 uORB Write  uORBTopic=vehicle_gps_position  selectInstance=vehicle_gps_position  MessageQueueLen=1
      settings: SourceProductBaseCode=PX4AUTOPILOTS
  Rate Transition : RateTransition
  Terminator : Terminator
  eph : Constant  Value=0.3  SampleTime=-1
  epv : Constant  Value=0.4  SampleTime=-1
  lat/lon in degE1 : Gain  Gain=1e7  OutDataTypeStr=Inherit: Inherit via back propagation
  lat/lon in degE7 : Gain  Gain=1e7  OutDataTypeStr=Inherit: Inherit via back propagation
  wires:
  Gain2/1 -> Bus Assignment/8
  lat/lon in degE7/1 -> Data Store Write/1, Bus Assignment/3
  Demux1/1 -> lat/lon in degE7/1
  Demux/3 -> Bus Assignment/11
  PX4 uORB Read/2 -> Bus Assignment/1
  Gain1/1 -> Data Type Conversion2/1
  Demux1/3 -> Altitude in mm/1
  Demux1/2 -> lat/lon in degE1/1
  Demux/1 -> Bus Assignment/9
  lat/lon in degE1/1 -> Data Store Write1/1, Bus Assignment/4
  Altitude in mm/1 -> Data Store Write2/1, Bus Assignment/5
  Data Type Conversion2/1 -> Demux/1
  Demux/2 -> Bus Assignment/10
  Bus Assignment/1 -> PX4 uORB Write/1
  "Number of satellites visible. If unknown, set to 255"/1 -> Bus Assignment/14
  Gain/1 -> Bus Assignment/6
  Gain3/1 -> Bus Assignment/7
  LLA/1 -> Demux1/1
  GndSpeed/1 -> Gain2/1
  Velocity/1 -> Gain1/1
  Course/1 -> Gain4/1
  Data Type Conversion1/1 -> Bus Assignment/12
  eph/1 -> Gain/1  "filter_eph"
  epv/1 -> Gain3/1  "filter_epv"
  Data Type Conversion3/1 -> Bus Assignment/13
  Gain4/1 -> Data Type Conversion1/1
  Constant3/1 -> Data Type Conversion3/1
  Rate Transition/1 -> Multiply/1
  Multiply/1 -> Bus Assignment/2
  PX4 uORB Read/1 -> Terminator/1
  Digital Clock/1 -> Rate Transition/1

== system px4_noGPS1/Position controller ==
  x : Inport
  x_d : Inport  Port=2
  y : Inport  Port=3
  y_d : Inport  Port=4
  Constant : Constant  Value=0
  Gain2 : Gain  Gain=0.01
  Gain4 : Gain  Gain=0.01
  Saturation1 : Saturate
  Saturation2 : Saturate
  Subsystem1 : Subsystem  mask{c=1, g=1}
      mask prompts: c "gain_1"; g "gain_2"
  Subsystem3 : Subsystem  mask{c=1, g=1}
      mask prompts: c "gain_1"; g "gain_2"
  q_x : Outport
  q_y : Outport  Port=2
  q_z : Outport  Port=3
  wires:
  Constant/1 -> q_z/1
  Gain2/1 -> Saturation1/1
  Saturation1/1 -> q_y/1
  Subsystem1/1(Out1) -> Gain2/1
  Saturation2/1 -> q_x/1
  Gain4/1 -> Saturation2/1
  Subsystem3/1(Out1) -> Gain4/1
  x_d/1 -> Subsystem3/2(In2)  "x_d"
  x/1 -> Subsystem3/1(In1)  "x"
  y/1 -> Subsystem1/1(In1)  "y"
  y_d/1 -> Subsystem1/2(In2)  "y_d"

== system px4_noGPS1/Subsystem ==
  Constant7 : Constant  Value=0
  Data Store Read54 : DataStoreRead  DataStoreName=position_flag  IndexOptions=Index vector (dialog)  Indices=1  OutputSizes=1
  Data Store Read55 : DataStoreRead  DataStoreName=pitch_desire  IndexOptions=Index vector (dialog)  Indices=1  OutputSizes=1
  Data Store Read56 : DataStoreRead  DataStoreName=roll_desire  IndexOptions=Index vector (dialog)  Indices=1  OutputSizes=1
  Mux7 : Mux  Inputs=2
  Switch3 : Switch  Criteria=u2 > Threshold  SaturateOnIntegerOverflow=off  InputSameDT=off
  des_pitch/roll : Outport
  wires:
  Switch3/1 -> des_pitch/roll/1
  Mux7/1 -> Switch3/1
  Constant7/1 -> Switch3/3
  Data Store Read55/1 -> Mux7/1
  Data Store Read54/1 -> Switch3/2
  Data Store Read56/1 -> Mux7/2

== system px4_noGPS1/Subsystem1 ==
  Enable : EnablePort
  Constant9 : Constant
  Data Store Write27 : DataStoreWrite  DataStoreName=t  IndexOptions=Index vector (dialog)  Indices=1  OutputSizes=1
  Discrete-Time Integrator : DiscreteIntegrator  SampleTime=-1  ICPrevOutput=DiscIntNeverNeededParam  ICPrevScaledInput=DiscIntNeverNeededParam
  wires:
  Constant9/1 -> Discrete-Time Integrator/1
  Discrete-Time Integrator/1 -> Data Store Write27/1

== system px4_noGPS1/Subsystem2 ==
  u : Inport
  Enable : EnablePort
  Data Store Write5 : DataStoreWrite  DataStoreName=d_x  IndexOptions=Index vector (dialog)  Indices=1  OutputSizes=1
  Data Store Write6 : DataStoreWrite  DataStoreName=d_y  IndexOptions=Index vector (dialog)  Indices=1  OutputSizes=1
  Demux : Demux  Outputs=2
  MATLAB Function5 : MATLAB Function  TreatAsAtomicUnit=on
  wires:
  Demux/2 -> Data Store Write6/1
  MATLAB Function5/1(y) -> Demux/1
  Demux/1 -> Data Store Write5/1
  u/1 -> MATLAB Function5/1(u)

== system px4_noGPS1/attitude_button ==
  Data Store Write28 : DataStoreWrite  DataStoreName=attitude_flag  IndexOptions=Index vector (dialog)  Indices=1  OutputSizes=1
  attitude_flag : Constant  OutDataTypeStr=boolean
  wires:
  attitude_flag/1 -> Data Store Write28/1

== system px4_noGPS1/observer_button ==
  Data Store Write28 : DataStoreWrite  DataStoreName=observer_flag  IndexOptions=Index vector (dialog)  Indices=1  OutputSizes=1
  observer_flag : Constant  Value=0  OutDataTypeStr=boolean
  wires:
  observer_flag/1 -> Data Store Write28/1

== system px4_noGPS1/position_button ==
  Data Store Write28 : DataStoreWrite  DataStoreName=position_flag  IndexOptions=Index vector (dialog)  Indices=1  OutputSizes=1
  position_flag : Constant  OutDataTypeStr=boolean
  wires:
  position_flag/1 -> Data Store Write28/1

== system px4_noGPS1/serial_button ==
  Data Store Write28 : DataStoreWrite  DataStoreName=serial_flag  IndexOptions=Index vector (dialog)  Indices=1  OutputSizes=1
  serial_flag : Constant  OutDataTypeStr=boolean
  wires:
  serial_flag/1 -> Data Store Write28/1

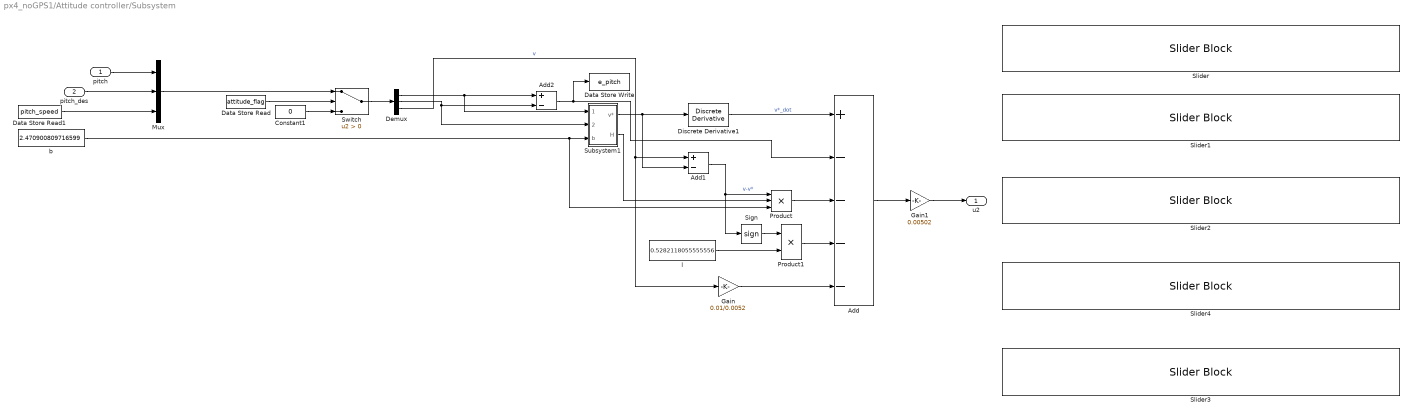
== system px4_noGPS1/Attitude controller/Subsystem ==
  pitch : Inport
  pitch_des : Inport  Port=2
  Add : Sum  Inputs=+----
  Add1 : Sum  Inputs=+-
  Add2 : Sum  Inputs=+-
  Constant1 : Constant  Value=0
  Data Store Read : DataStoreRead  DataStoreName=attitude_flag  IndexOptions=Index vector (dialog)  Indices=1  OutputSizes=1
  Data Store Read1 : DataStoreRead  DataStoreName=pitch_speed  IndexOptions=Index vector (dialog)  Indices=1  OutputSizes=1
  Data Store Write : DataStoreWrite  DataStoreName=e_pitch  IndexOptions=Index vector (dialog)  Indices=1  OutputSizes=1
  Demux : Demux  Outputs=3
  Discrete Derivative1 : simulink/Discrete/Discrete Derivative  gainval=1.0  ICPrevScaledInput=0.0  OutMin=[]  OutMax=[]  OutDataType=fixdt(1, 16)  OutScaling=2^-10  DoSatur=off
  Gain : Gain  Gain=0.01/0.0052
  Gain1 : Gain  Gain=0.00502
  Mux : Mux  Inputs=3
  Product : Product  Inputs=3
  Product1 : Product
  Sign : Signum
  Slider : SliderBlock  ScaleMax=20
  Slider1 : SliderBlock  ScaleMax=20
  Slider2 : SliderBlock  ScaleMin=2  ScaleMax=10
  Slider3 : SliderBlock  ScaleMax=20
  Slider4 : SliderBlock  ScaleMax=10
  Subsystem1 : Subsystem
  Switch : Switch  Criteria=u2 > Threshold  SaturateOnIntegerOverflow=off  InputSameDT=off
  b : Constant  Value=2.470900809716599
  l : Constant  Value=0.5282118055555556
  u2 : Outport
  wires:
  Product/1 -> Add/3
  Add1/1 -> Sign/1, Product/1  "v-v*"
  Demux/3 -> Gain/1, Add1/1  "v"
  pitch/1 -> Mux/1
  Discrete Derivative1/1 -> Add/1  "v*_dot"
  l/1 -> Product1/2
  b/1 -> Subsystem1/3(b), Product/3
  Subsystem1/2(H) -> Product/2
  Subsystem1/1(v*) -> Add1/2, Discrete Derivative1/1
  Sign/1 -> Product1/1
  Add/1 -> Gain1/1
  pitch_des/1 -> Mux/2
  Add2/1 -> Data Store Write/1, Add/2
  Product1/1 -> Add/4
  Gain/1 -> Add/5
  Gain1/1 -> u2/1
  Data Store Read/1 -> Switch/2
  Switch/1 -> Demux/1
  Constant1/1 -> Switch/3
  Mux/1 -> Switch/1
  Demux/1 -> Subsystem1/1(pitch), Add2/1
  Demux/2 -> Subsystem1/2(pitch_des), Add2/2
  Data Store Read1/1 -> Mux/3

== system px4_noGPS1/Attitude controller/Subsystem1 ==
  roll : Inport
  roll_des : Inport  Port=2
  Add : Sum  Inputs=+----
  Add1 : Sum  Inputs=+-
  Add2 : Sum  Inputs=+-
  Discrete Derivative : simulink/Discrete/Discrete Derivative  gainval=1.0  ICPrevScaledInput=0.0  OutMin=[]  OutMax=[]  OutDataType=fixdt(1, 16)  OutScaling=2^-10  DoSatur=off
  Discrete Derivative1 : simulink/Discrete/Discrete Derivative  gainval=1.0  ICPrevScaledInput=0.0  OutMin=[]  OutMax=[]  OutDataType=fixdt(1, 16)  OutScaling=2^-10  DoSatur=off
  Gain : Gain  Gain=0.01/0.00478
  Gain1 : Gain  Gain=0.00478
  Product : Product  Inputs=3
  Product1 : Product
  Sign : Signum
  Subsystem1 : Subsystem
  b : Constant
  l : Constant  Value=0
  u2 : Outport
  wires:
  Product/1 -> Add/3
  Add1/1 -> Sign/1, Product/1  "v-v*"
  Discrete Derivative/1 -> Gain/1, Add1/1  "v"
  roll/1 -> Discrete Derivative/1, Subsystem1/1(roll), Add2/1
  Discrete Derivative1/1 -> Add/1  "v*_dot"
  l/1 -> Product1/2
  b/1 -> Subsystem1/3(b), Product/3
  Subsystem1/2(H) -> Product/2
  Subsystem1/1(v*) -> Add1/2, Discrete Derivative1/1
  Sign/1 -> Product1/1
  Add/1 -> Gain1/1
  roll_des/1 -> Subsystem1/2(roll_des), Add2/2
  Add2/1 -> Add/2
  Product1/1 -> Add/4
  Gain/1 -> Add/5
  Gain1/1 -> u2/1

== system px4_noGPS1/Attitude controller/Subsystem2 ==
  u : Inport
  Add : Sum
  Add1 : Sum  Inputs=+-
  Add2 : Sum
  Divide : Product  Inputs=*/
  Gain : Gain  Gain=0.5
  Gain1 : Gain  Gain=0.5
  Gain2 : Gain  Gain=sqrt(pi)/2
  MATLAB Function : MATLAB Function  TreatAsAtomicUnit=on
  Product : Product
  Product2 : Product
  Sign : Signum
  lower bound : Constant  Value=0.5
  upper bound : Constant  Value=0.5
  sat_u : Outport
  wires:
  Add2/1 -> Product2/1, Divide/2  "tm"
  lower bound/1 -> Add1/2, Add/2
  u/1 -> Sign/1, Gain2/1
  Sign/1 -> Product/2
  Add1/1 -> Gain1/1
  Product/1 -> Add2/2
  upper bound/1 -> Add/1, Add1/1
  Gain1/1 -> Product/1
  Gain2/1 -> Divide/1
  Gain/1 -> Add2/1
  Add/1 -> Gain/1
  Divide/1 -> MATLAB Function/1(u)
  MATLAB Function/1(y) -> Product2/2
  Product2/1 -> sat_u/1
